simulink model "microgrid"  (R2021b)
settings: Solver=ode23tb  StartTime=0.0  StopTime=1  FixedStep=5e-6  RelTol=1e-3  EnableMultiTasking=on
PreLoadFcn:
  | % ---- microgrid : PreLoadFcn -------------------------------------
  | % Loads every base-workspace parameter this model needs.
  | %   SolarPVMPPTBoostData.mlx : PV array, boost converter, MPPT controller
  | %   microgridParams.m        : bus, battery, grid, drain, droop  (struct mg)
  | try
  |     mgDir = fileparts(which('microgrid'));
  |     if ~isempty(mgDir) && ~contains([path pathsep], [mgDir pathsep])
  |         addpath(mgDir);
  |     end
  |     evalc('SolarPVMPPTBoostData');
  |     microgridParams;
  |     clear mgDir
  |     disp('microgrid: parameters loaded (SolarPVMPPTBoostData + microgridParams).');
  | catch mgErr
  |     warning('microgrid:paramLoadFailed', ...
  |             'Could not load model parameters: %s', mgErr.message);
  |     clear mgErr
  | end
values from neighbouring files (symbols this model uses):
  mg = evalin('base','mg')    [microgridCheck.m]    (also in microgridParams.m = struct(); microgridScenario.m)
undefined symbols (not defined in the file or in its folder): boostController, dcVoltage, Ion, Lithium, sensor, solarPanel, solarPlant
libraries: powerlib_extras x46, fl_lib x12, simulink x8, nesl_utility x8, spsSeriesRLCBranchLib x7, spsCurrentMeasurementLib x7, spsGroundLib x6, spsVoltageMeasurementLib x6, spsIGBTDiodeLib x4, spsVariableResistorLib x4, slpidlib x4, ee_lib x3
(part 2 of 3)

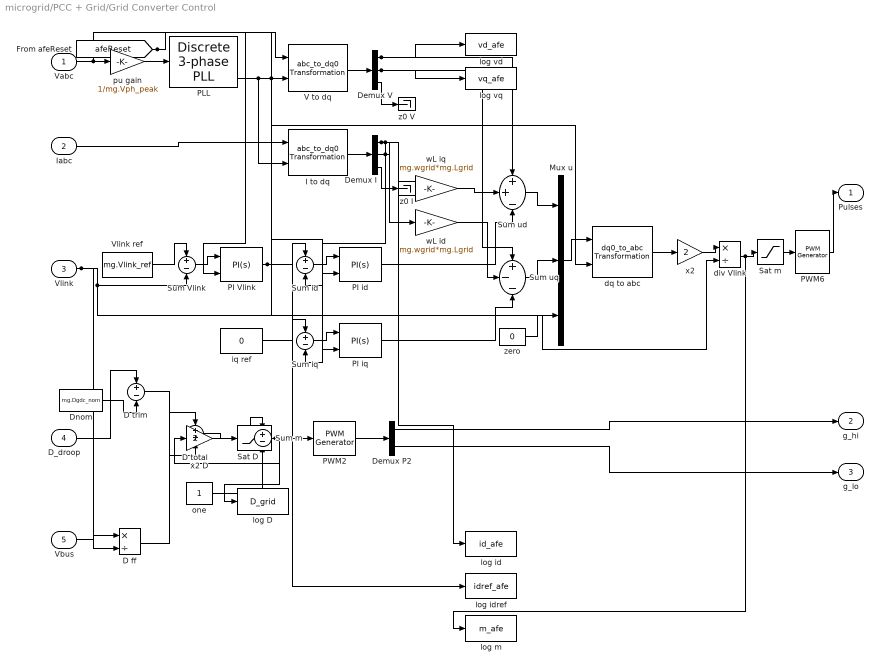
== system microgrid/PCC + Grid/Grid Converter Control ==
  Vabc : Inport
  Iabc : Inport  Port=2
  Vlink : Inport  Port=3
  D_droop : Inport  Port=4
  Vbus : Inport  Port=5
  D ff : Product  Inputs=*/
  D total : Sum
  D trim : Sum  Inputs=+-
  Demux I : Demux  Outputs=3
  Demux P2 : Demux  Outputs=2
  Demux V : Demux  Outputs=3
  Dnom : Constant  Value=mg.Dgdc_nom
  I to dq : powerlib_extras/Measurements/abc_to_dq0 Transformation
      settings: SourceProductBaseCode=PS
  Mux u : Mux  Inputs=3
  PI Vlink : slpidlib/PID Controller  Controller=PI  Form=Parallel  TimeDomain=Continuous-time  UseExternalTs=off  SampleTime=-1  IntegratorMethod=Forward Euler  FilterMethod=Forward Euler  ControllerParametersSource=internal  P=mg.Kp_v_afe  I=mg.Ki_v_afe  D=0  UseFilter=on  N=100  TunerSelectOption=Transfer Function Based (PID Tuner App)  InitialConditionSource=internal  InitialConditionForIntegrator=0  InitialConditionForFilter=0  DifferentiatorICPrevScaledInput=0  ExternalReset=level  TrackingMode=off  Kt=1  LimitOutput=on  SatLimitsSource=internal  UpperSaturationLimit=mg.Id_max  LowerSaturationLimit=-mg.Id_max  LinearizeAsGain=on  AntiWindupMode=clamping  Kb=1  POutMin=[]  POutMax=[]  IOutMin=[]  IOutMax=[]  DOutMin=[]  DOutMax=[]  NOutMin=[]  NOutMax=[]  SumOutMin=[]  SumOutMax=[]  SaturationOutMin=[]  SaturationOutMax=[]  PParamMin=[]  PParamMax=[]  IParamMin=[]  IParamMax=[]  DParamMin=[]  DParamMax=[]  NParamMin=[]  NParamMax=[]  KbParamMin=[]  KbParamMax=[]  KtParamMin=[]  KtParamMax=[]  KbOutMin=[]  KbOutMax=[]  KtOutMin=[]  KtOutMax=[]  IntegratorOutMin=[]  IntegratorOutMax=[]  FilterOutMin=[]  FilterOutMax=[]  SumI1OutMin=[]  SumI1OutMax=[]  SumI2OutMin=[]  SumI2OutMax=[]  SumI3OutMin=[]  SumI3OutMax=[]  SumI4OutMin=[]  SumI4OutMax=[]  SumDOutMin=[]  SumDOutMax=[]  DifferentiatorOutMin=[]  DifferentiatorOutMax=[]  FilterDiffOutCoefMin=[]  FilterDiffOutCoefMax=[]  ReciprocalOutMin=[]  ReciprocalOutMax=[]  SumDenOutMin=[]  SumDenOutMax=[]  SumNumOutMin=[]  SumNumOutMax=[]  DivideOutMin=[]  DivideOutMax=[]  UdiffTsProdOutMin=[]  UdiffTsProdOutMax=[]  NTsProdOutMin=[]  NTsProdOutMax=[]  UintegralTsProdOutMin=[]  UintegralTsProdOutMax=[]  UngainTsProdOutMin=[]  UngainTsProdOutMax=[]  FilterDenConstantOutDataTypeStr=Inherit: Inherit via back propagation  FilterDenConstantOutMin=[]  FilterDenConstantOutMax=[]  PCopyOutDataTypeStr=Inherit: Inherit via back propagation  PCopyOutMin=[]  PCopyOutMax=[]  NCopyOutDataTypeStr=Inherit: Inherit via back propagation  NCopyOutMin=[]  NCopyOutMax=[]  IntegratorContinuousStateAttributes=''  IntegratorStateMustResolveToSignalObject=off  IntegratorRTWStateStorageClass=Auto  FilterContinuousStateAttributes=''  FilterStateMustResolveToSignalObject=off  FilterRTWStateStorageClass=Auto  ParallelPVariant=InternalParameters  IdealPVariant=Disabled  IVariant=InternalParameters  DVariant=Disabled  IntegratorVariant=Continuous  SatVariant=Enabled  AWVariant=ContClampingParallel  PCopyVariant=Disabled  TRVariant=Disabled  FdbkBlocksVariant=Forward  IdealPFdbkVariant=Disabled  SatFdbkVariant=Disabled  DerivativeFilterVariant=Disabled  NVariant=Disabled  NCopyVariant=Disabled_SignalSpec  FilterICVariant=Disabled  IntegratorICVariant=InternalICs  ExternalResetVariant=ExternalReset  TRSumVariant=Passthrough  SumFdbkVariant=Disabled  SumVariant=Sum_PI  TsampFilterVariant=InternalTs  TsampNgainVariant=Passthrough  TsampIntegralVariant=Passthrough  ExternalSaturationOutDataTypeStr=Inherit: Same as second input
  PI id : slpidlib/PID Controller  Controller=PI  Form=Parallel  TimeDomain=Continuous-time  UseExternalTs=off  SampleTime=-1  IntegratorMethod=Forward Euler  FilterMethod=Forward Euler  ControllerParametersSource=internal  P=mg.Kp_i_afe  I=mg.Ki_i_afe  D=0  UseFilter=on  N=100  TunerSelectOption=Transfer Function Based (PID Tuner App)  InitialConditionSource=internal  InitialConditionForIntegrator=0  InitialConditionForFilter=0  DifferentiatorICPrevScaledInput=0  ExternalReset=level  TrackingMode=off  Kt=1  LimitOutput=on  SatLimitsSource=internal  UpperSaturationLimit=mg.Vph_peak  LowerSaturationLimit=-mg.Vph_peak  LinearizeAsGain=on  AntiWindupMode=clamping  Kb=1  POutMin=[]  POutMax=[]  IOutMin=[]  IOutMax=[]  DOutMin=[]  DOutMax=[]  NOutMin=[]  NOutMax=[]  SumOutMin=[]  SumOutMax=[]  SaturationOutMin=[]  SaturationOutMax=[]  PParamMin=[]  PParamMax=[]  IParamMin=[]  IParamMax=[]  DParamMin=[]  DParamMax=[]  NParamMin=[]  NParamMax=[]  KbParamMin=[]  KbParamMax=[]  KtParamMin=[]  KtParamMax=[]  KbOutMin=[]  KbOutMax=[]  KtOutMin=[]  KtOutMax=[]  IntegratorOutMin=[]  IntegratorOutMax=[]  FilterOutMin=[]  FilterOutMax=[]  SumI1OutMin=[]  SumI1OutMax=[]  SumI2OutMin=[]  SumI2OutMax=[]  SumI3OutMin=[]  SumI3OutMax=[]  SumI4OutMin=[]  SumI4OutMax=[]  SumDOutMin=[]  SumDOutMax=[]  DifferentiatorOutMin=[]  DifferentiatorOutMax=[]  FilterDiffOutCoefMin=[]  FilterDiffOutCoefMax=[]  ReciprocalOutMin=[]  ReciprocalOutMax=[]  SumDenOutMin=[]  SumDenOutMax=[]  SumNumOutMin=[]  SumNumOutMax=[]  DivideOutMin=[]  DivideOutMax=[]  UdiffTsProdOutMin=[]  UdiffTsProdOutMax=[]  NTsProdOutMin=[]  NTsProdOutMax=[]  UintegralTsProdOutMin=[]  UintegralTsProdOutMax=[]  UngainTsProdOutMin=[]  UngainTsProdOutMax=[]  FilterDenConstantOutDataTypeStr=Inherit: Inherit via back propagation  FilterDenConstantOutMin=[]  FilterDenConstantOutMax=[]  PCopyOutDataTypeStr=Inherit: Inherit via back propagation  PCopyOutMin=[]  PCopyOutMax=[]  NCopyOutDataTypeStr=Inherit: Inherit via back propagation  NCopyOutMin=[]  NCopyOutMax=[]  IntegratorContinuousStateAttributes=''  IntegratorStateMustResolveToSignalObject=off  IntegratorRTWStateStorageClass=Auto  FilterContinuousStateAttributes=''  FilterStateMustResolveToSignalObject=off  FilterRTWStateStorageClass=Auto  ParallelPVariant=InternalParameters  IdealPVariant=Disabled  IVariant=InternalParameters  DVariant=Disabled  IntegratorVariant=Continuous  SatVariant=Enabled  AWVariant=ContClampingParallel  PCopyVariant=Disabled  TRVariant=Disabled  FdbkBlocksVariant=Forward  IdealPFdbkVariant=Disabled  SatFdbkVariant=Disabled  DerivativeFilterVariant=Disabled  NVariant=Disabled  NCopyVariant=Disabled_SignalSpec  FilterICVariant=Disabled  IntegratorICVariant=InternalICs  ExternalResetVariant=ExternalReset  TRSumVariant=Passthrough  SumFdbkVariant=Disabled  SumVariant=Sum_PI  TsampFilterVariant=InternalTs  TsampNgainVariant=Passthrough  TsampIntegralVariant=Passthrough  ExternalSaturationOutDataTypeStr=Inherit: Same as second input
  PI iq : slpidlib/PID Controller  Controller=PI  Form=Parallel  TimeDomain=Continuous-time  UseExternalTs=off  SampleTime=-1  IntegratorMethod=Forward Euler  FilterMethod=Forward Euler  ControllerParametersSource=internal  P=mg.Kp_i_afe  I=mg.Ki_i_afe  D=0  UseFilter=on  N=100  TunerSelectOption=Transfer Function Based (PID Tuner App)  InitialConditionSource=internal  InitialConditionForIntegrator=0  InitialConditionForFilter=0  DifferentiatorICPrevScaledInput=0  ExternalReset=level  TrackingMode=off  Kt=1  LimitOutput=on  SatLimitsSource=internal  UpperSaturationLimit=mg.Vph_peak  LowerSaturationLimit=-mg.Vph_peak  LinearizeAsGain=on  AntiWindupMode=clamping  Kb=1  POutMin=[]  POutMax=[]  IOutMin=[]  IOutMax=[]  DOutMin=[]  DOutMax=[]  NOutMin=[]  NOutMax=[]  SumOutMin=[]  SumOutMax=[]  SaturationOutMin=[]  SaturationOutMax=[]  PParamMin=[]  PParamMax=[]  IParamMin=[]  IParamMax=[]  DParamMin=[]  DParamMax=[]  NParamMin=[]  NParamMax=[]  KbParamMin=[]  KbParamMax=[]  KtParamMin=[]  KtParamMax=[]  KbOutMin=[]  KbOutMax=[]  KtOutMin=[]  KtOutMax=[]  IntegratorOutMin=[]  IntegratorOutMax=[]  FilterOutMin=[]  FilterOutMax=[]  SumI1OutMin=[]  SumI1OutMax=[]  SumI2OutMin=[]  SumI2OutMax=[]  SumI3OutMin=[]  SumI3OutMax=[]  SumI4OutMin=[]  SumI4OutMax=[]  SumDOutMin=[]  SumDOutMax=[]  DifferentiatorOutMin=[]  DifferentiatorOutMax=[]  FilterDiffOutCoefMin=[]  FilterDiffOutCoefMax=[]  ReciprocalOutMin=[]  ReciprocalOutMax=[]  SumDenOutMin=[]  SumDenOutMax=[]  SumNumOutMin=[]  SumNumOutMax=[]  DivideOutMin=[]  DivideOutMax=[]  UdiffTsProdOutMin=[]  UdiffTsProdOutMax=[]  NTsProdOutMin=[]  NTsProdOutMax=[]  UintegralTsProdOutMin=[]  UintegralTsProdOutMax=[]  UngainTsProdOutMin=[]  UngainTsProdOutMax=[]  FilterDenConstantOutDataTypeStr=Inherit: Inherit via back propagation  FilterDenConstantOutMin=[]  FilterDenConstantOutMax=[]  PCopyOutDataTypeStr=Inherit: Inherit via back propagation  PCopyOutMin=[]  PCopyOutMax=[]  NCopyOutDataTypeStr=Inherit: Inherit via back propagation  NCopyOutMin=[]  NCopyOutMax=[]  IntegratorContinuousStateAttributes=''  IntegratorStateMustResolveToSignalObject=off  IntegratorRTWStateStorageClass=Auto  FilterContinuousStateAttributes=''  FilterStateMustResolveToSignalObject=off  FilterRTWStateStorageClass=Auto  ParallelPVariant=InternalParameters  IdealPVariant=Disabled  IVariant=InternalParameters  DVariant=Disabled  IntegratorVariant=Continuous  SatVariant=Enabled  AWVariant=ContClampingParallel  PCopyVariant=Disabled  TRVariant=Disabled  FdbkBlocksVariant=Forward  IdealPFdbkVariant=Disabled  SatFdbkVariant=Disabled  DerivativeFilterVariant=Disabled  NVariant=Disabled  NCopyVariant=Disabled_SignalSpec  FilterICVariant=Disabled  IntegratorICVariant=InternalICs  ExternalResetVariant=ExternalReset  TRSumVariant=Passthrough  SumFdbkVariant=Disabled  SumVariant=Sum_PI  TsampFilterVariant=InternalTs  TsampNgainVariant=Passthrough  TsampIntegralVariant=Passthrough  ExternalSaturationOutDataTypeStr=Inherit: Same as second input
  PLL : powerlib_extras/Discrete  Control Blocks/Discrete 3-phase PLL  Fmin=0.8*mg.fgrid  Par_Init=[0 mg.fgrid]  ParK=[ 180 3200 1 ]  Ts=mg.Ts_pll  AGC=on
      settings: SourceProductBaseCode=PS
  PWM2 : powerlib_extras/Control  Blocks/PWM Generator  GeneratorMode="1-arm  bridge (2 pulses)"  Fc=mg.fsw_gdc  Internal=off  mIndex=0.4  Freq=mg.fgrid  Phase=0
      settings: SourceProductBaseCode=PS
  PWM6 : powerlib_extras/Control  Blocks/PWM Generator  GeneratorMode="3-arm  bridge (6 pulses)"  Fc=mg.fsw_afe  Internal=off  mIndex=0.4  Freq=mg.fgrid  Phase=0
      settings: SourceProductBaseCode=PS
  Sat D : Saturate  UpperLimit=mg.Dgdc_max  LowerLimit=mg.Dgdc_min
  Sat m : Saturate  UpperLimit=1  LowerLimit=-1
  Sum Vlink : Sum  Inputs=+-
  Sum id : Sum  Inputs=+-
  Sum iq : Sum  Inputs=+-
  Sum m : Sum  Inputs=+-
  Sum ud : Sum  Inputs=++-
  Sum uq : Sum  Inputs=+--
  V to dq : powerlib_extras/Measurements/abc_to_dq0 Transformation
      settings: SourceProductBaseCode=PS
  Vlink ref : Constant  Value=mg.Vlink_ref
  div Vlink : Product  Inputs=*/
  dq to abc : powerlib_extras/Measurements/dq0_to_abc Transformation
      settings: SourceProductBaseCode=PS
  iq ref : Constant  Value=0
  log D : ToWorkspace  VariableName=D_grid  SampleTime=-1
      settings: Decimation=20
  log id : ToWorkspace  VariableName=id_afe  SampleTime=-1
      settings: Decimation=20
  log idref : ToWorkspace  VariableName=idref_afe  SampleTime=-1
      settings: Decimation=20
  log m : ToWorkspace  VariableName=m_afe  SampleTime=-1
      settings: Decimation=20
  log vd : ToWorkspace  VariableName=vd_afe  SampleTime=-1
      settings: Decimation=20
  log vq : ToWorkspace  VariableName=vq_afe  SampleTime=-1
      settings: Decimation=20
  one : Constant
  pu gain : Gain  Gain=1/mg.Vph_peak
  wL id : Gain  Gain=mg.wgrid*mg.Lgrid
  wL iq : Gain  Gain=mg.wgrid*mg.Lgrid
  x2 : Gain  Gain=2
  x2 D : Gain  Gain=2
  z0 I : Terminator
  z0 V : Terminator
  zero : Constant  Value=0
  Pulses : Outport
  g_hi : Outport  Port=2
  g_lo : Outport  Port=3
  wires:
  Vabc/1 -> pu gain/1, V to dq/1
  pu gain/1 -> PLL/1
  PLL/3 -> V to dq/2, dq to abc/2, I to dq/2
  Iabc/1 -> I to dq/1
  V to dq/1 -> Demux V/1
  I to dq/1 -> Demux I/1
  Vlink ref/1 -> Sum Vlink/1
  Vlink/1 -> Sum Vlink/2, div Vlink/2, D ff/2
  Sum Vlink/1 -> PI Vlink/1
  PI Vlink/1 -> Sum id/1, log idref/1
  Demux I/1 -> Sum id/2, wL id/1, log id/1
  iq ref/1 -> Sum iq/1
  Demux I/2 -> Sum iq/2, wL iq/1
  Sum id/1 -> PI id/1
  Sum iq/1 -> PI iq/1
  Demux V/1 -> Sum ud/1, log vd/1
  wL iq/1 -> Sum ud/2
  PI id/1 -> Sum ud/3
  Demux V/2 -> Sum uq/1, log vq/1
  wL id/1 -> Sum uq/2
  PI iq/1 -> Sum uq/3
  Sum ud/1 -> Mux u/1
  Sum uq/1 -> Mux u/2
  zero/1 -> Mux u/3
  Mux u/1 -> dq to abc/1
  dq to abc/1 -> x2/1
  x2/1 -> div Vlink/1
  div Vlink/1 -> Sat m/1, log m/1
  Sat m/1 -> PWM6/1
  PWM6/1 -> Pulses/1
  x2 D/1 -> Sum m/1
  one/1 -> Sum m/2
  Sum m/1 -> PWM2/1
  PWM2/1 -> Demux P2/1
  Demux P2/1 -> g_hi/1
  Demux P2/2 -> g_lo/1
  Vbus/1 -> D ff/1
  D_droop/1 -> D trim/1
  Dnom/1 -> D trim/2
  D ff/1 -> D total/1
  D trim/1 -> D total/2
  D total/1 -> Sat D/1
  Sat D/1 -> x2 D/1, log D/1
  Demux V/3 -> z0 V/1
  Demux I/3 -> z0 I/1
  [afeReset] -> PI Vlink/2, PI id/2, PI iq/2

== system microgrid/PV + Boost/AC Current Sensor2 ==
  Current Sensor : fl_lib/Electrical/Electrical Sensors/Current Sensor
  PS-Simulink Converter : nesl_utility/PS-Simulink Converter  PhysicalDomain=network_engine_domain  SubClassName=ps_output  LeftPortType=input  RightPortType=output  PseudoPeriodic=off  Frequencies=[]  Unit=1  AffineConversion=off
      settings: SourceProductBaseCode=PW,SS
  Sensor dynamics : TransferFcn  Numerator=1  Denominator=[1/sensor.samplingFreq 1]
  - : PMIOPort  Side=Left
  + : PMIOPort  Port=2  Side=Right
  tag scope: Iload=global
  wires:
  PS-Simulink Converter/1 -> Sensor dynamics/1
  Sensor dynamics/1 -> [Iload]
  connections:
  Current Sensor/RConn1 -- PS-Simulink Converter/LConn1
  +/RConn1 -- Current Sensor/LConn1
  Current Sensor/RConn2 -- -/RConn1

== system microgrid/PV + Boost/Boost Converter ==
  m : Inport
  AC Current Sensor1 : Subsystem
      mask Display: disp('i');
  DC Bus Capacitor : fl_lib/Electrical/Electrical Elements/Capacitor  c=mg.Cbus F  r=1e-6 Ohm  g=0 1/Ohm  i_specify=off  i_priority=None  i=0 A  i_nominal_specify=off  i_nominal_unit=A  i_nominal_value=1  v_specify=off  v_priority=None  v=0 V  v_nominal_specify=off  v_nominal_unit=V  v_nominal_value=1  vc_specify=on  vc_priority=High  vc=mg.Vbus_nom V  vc_nominal_specify=off  vc_nominal_unit=V  vc_nominal_value=1
  Diode : fl_lib/Electrical/Electrical Elements/Diode  Vf=0.6 V  Ron=0.3 Ohm  Goff=1e-8 1/Ohm  i_specify=off  i_priority=None  i=0 A  i_nominal_specify=off  i_nominal_unit=A  i_nominal_value=1  v_specify=off  v_priority=None  v=0 V  v_nominal_specify=off  v_nominal_unit=V  v_nominal_value=1
  Gain : Gain  Gain=5
  "IGBT (Ideal, Switching)1" : ee_lib/Semiconductors & Converters/IGBT (Ideal, Switching)  Vf=0.8 V  Ron=0.001 Ohm  Goff=1e-5 1/Ohm  Vth=2.5 V  diode_param=1  diode_Vf=0.8 V  diode_Ron=0.001 Ohm  diode_Goff=1e-5 1/Ohm  diode_C=50e-9 F  diode_iRM=-235 A  diode_iF=300 A  diode_idot=-50 A/us  diode_trr_param=1  diode_trr_factor=3  diode_trr=15 us  diode_Qrr=1500 s*uA  thermal_loss_option=ee.enum.converters.thermalLossOption.constantvalues  Von_data=[0, .1, .6, .8, 1, 1.3, 1.6, 2, 2.4; 0, .1, .7, 1, 1.2, 1.5, 1.9, 2.4, 2.8] V  Tj=[298.15, 398.15] K  Iout_data=[0, .1, 1, 5, 10, 20, 40, 70, 100] A  Eon_data=[0, .0024, .024, .12, .2, .48, 1.04, 2.16, 3.24; 0, .003, .03, .15, .25, .6, 1.3, 2.7, 4.05] * 1e-3 J  Eoff_data=[0, .0007, .0066, .033, .066, .17, .33, .83, 1.5; 0, .001, .01, .05, .1, .25, .5, 1.2, 2.2] * 1e-3 J  Tj_loss=[298.15, 398.15] K  Iout_data_loss=[0, .1, 1, 5, 10, 20, 40, 70, 100] A  Eon_scalar=22.86e-3 J  Eoff_scalar=17.14e-3 J  Voff=300 V  Iout_scalar=600 A  diodeModelType=ee.enum.converters.diodeModelType.pwl  diodeTableType=ee.enum.diode.tableType.IfMat  diode_IfMat=[.07, .12, .19, 1.75, 4.24, 7.32, 11.2; .16, .3, .72, 2.14, 4.02, 6.35, 9.12] A  diode_VfMat=[.9, 1.15, 1.25, 1.5, 1.75, 2.17, 2.6, 2.85; .58, .68, .75, 1.1, 1.38, 1.77, 2.27, 2.7] V  diode_TjVec=[25, 125] degC  diode_VfVec=[.5, .7, .9, 1.3, 1.7, 2.1, 2.5] V  diode_IfVec=[.1, .2, .5, 1, 2, 4, 7, 10] A  diode_Vr=-600 V  diode_Ls=150 nH  diode_Erec=0.03 J  thermal_network_parameterization=ee.enum.thermalNetworkTopology.external  Rth=[.08, .5] K/W  Rth_Cauer=[.08, .1, .5] K/W  Rth_Foster=[.08, .14, .22, .16] K/W  thermal_mass_parameterization=ee.enum.thermalNetwork.timeconstant  thermal_mass=[.01, .5] J/K  thermal_mass_Cauer=[.01, .1, .5] J/K  thermal_mass_Foster=[.001, .005, .05, .5] J/K  thermal_time_constant=[.001, .2] s  thermal_time_constant_Cauer=[.001, .1, .2] s  thermal_time_constant_Foster=[7e-05, .0007, .01, .08] s  thermal_mass_initial_temperatures=[25, 25] degC  thermal_mass_initial_temperatures_Cauer=[25, 25, 25] degC  junction_thermal_mass=0.01 J/K  steadyState_Foster=simscape.enum.onoff.on  Tvec_initial_Foster=[25, 25, 25, 25] degC  no_thermal_network=0  junction_temperature_specify=off  junction_temperature_priority=None  junction_temperature=25 degC  junction_temperature_nominal_specify=off  junction_temperature_nominal_unit=degC  junction_temperature_nominal_value=1  vT_specify=off  vT_priority=None  vT=0 V  vT_nominal_specify=off  vT_nominal_unit=V  vT_nominal_value=1  Qj_specify=off  Qj_priority=None  Qj=0 W  Qj_nominal_specify=off  Qj_nominal_unit=W  Qj_nominal_value=1
  MPPT Inductor : ee_lib/Passive/Inductor  l=boost.inductor H  L_tol=5  enable_L_tol=0  tol_distribution=1  nSigma=4  r=boost.inductorResistance Ohm  g=1e-9 1/Ohm  enable_operating_limits=0  operating_limit_action=2  max_working_current=1 A  power_rating=1 W  enable_faults=0  fault_action=simscape.enum.assert.action.none  lambdaPercent=50  k_faulted=0.9999  turnsShort=0  openCct=0  groundShort=0  groundShortG=0 1/Ohm  tau_fault=1e-3 s  enable_temporal_fault=0  t_fault=1 s  enable_behavioral_fault=0  max_permissible_voltage=100 V  n_fail_on_voltage=1  max_permissible_current=1 A  t_fail_on_current=1 s  i_L_specify=on  i_L_priority=High  i_L=0 A  i_L_nominal_specify=off  i_L_nominal_unit=A  i_L_nominal_value=1
  Simulink-PS Converter : nesl_utility/Simulink-PS Converter  PhysicalDomain=network_engine_domain  SubClassName=ps_input  LeftPortType=input  RightPortType=output  PseudoPeriodic=off  Frequencies=[]  NoiseDistribution=none  NoiseParameters=[]  Unit=1  AffineConversion=off  FilteringAndDerivatives=provide  SimscapeFilterOrder=1  InputFilterTimeConstant=0.001  UdotUserProvided=0
      settings: SourceProductBaseCode=PW,SS
  + : PMIOPort  Side=Left
  P : PMIOPort  Port=2  Side=Right
  N : PMIOPort  Port=3  Side=Right
  - : PMIOPort  Port=4  Side=Left
  wires:
  m/1 -> Gain/1
  Gain/1 -> Simulink-PS Converter/1
  connections:
  MPPT Inductor/LConn1 -- AC Current Sensor1/LConn1
  N/RConn1 -- DC Bus Capacitor/RConn1 -- "IGBT (Ideal, Switching)1"/RConn2 -- -/RConn1
  AC Current Sensor1/RConn1 -- +/RConn1
  "IGBT (Ideal, Switching)1"/LConn1 -- Simulink-PS Converter/RConn1
  MPPT Inductor/RConn1 -- "IGBT (Ideal, Switching)1"/RConn1 -- Diode/LConn1
  DC Bus Capacitor/LConn1 -- Diode/RConn1 -- P/RConn1

== system microgrid/PV + Boost/DC Current Sensor ==
  Current Sensor : fl_lib/Electrical/Electrical Sensors/Current Sensor
      settings: LogSimulationData=on
  PS-Simulink Converter : nesl_utility/PS-Simulink Converter  PhysicalDomain=network_engine_domain  SubClassName=ps_output  LeftPortType=input  RightPortType=output  PseudoPeriodic=off  Frequencies=[]  Unit=1  AffineConversion=off
      settings: SourceProductBaseCode=PW,SS
  Sensor dynamics : TransferFcn  Numerator=1  Denominator=[1/sensor.samplingFreq 1]
  - : PMIOPort  Side=Left
  + : PMIOPort  Port=2  Side=Right
  tag scope: Ipv=global
  wires:
  PS-Simulink Converter/1 -> Sensor dynamics/1
  Sensor dynamics/1 -> [Ipv]
  connections:
  Current Sensor/RConn2 -- -/RConn1
  +/RConn1 -- Current Sensor/LConn1
  Current Sensor/RConn1 -- PS-Simulink Converter/LConn1

== system microgrid/PV + Boost/DC Output Voltage Sensor ==
  PS-Simulink Converter : nesl_utility/PS-Simulink Converter  PhysicalDomain=network_engine_domain  SubClassName=ps_output  LeftPortType=input  RightPortType=output  PseudoPeriodic=off  Frequencies=[]  Unit=1  AffineConversion=off
      settings: SourceProductBaseCode=PW,SS
  Sensor dynamics : TransferFcn  Numerator=1  Denominator=[1/sensor.samplingFreq 1]
  Voltage Sensor : fl_lib/Electrical/Electrical Sensors/Voltage Sensor
  - : PMIOPort  Side=Left
  + : PMIOPort  Port=2  Side=Right
  tag scope: Vo=global
  wires:
  PS-Simulink Converter/1 -> Sensor dynamics/1
  Sensor dynamics/1 -> [Vo]
  connections:
  Voltage Sensor/RConn2 -- -/RConn1
  Voltage Sensor/RConn1 -- PS-Simulink Converter/LConn1
  Voltage Sensor/LConn1 -- +/RConn1

== system microgrid/PV + Boost/DC Voltage Sensor ==
  PS-Simulink Converter : nesl_utility/PS-Simulink Converter  PhysicalDomain=network_engine_domain  SubClassName=ps_output  LeftPortType=input  RightPortType=output  PseudoPeriodic=off  Frequencies=[]  Unit=1  AffineConversion=off
      settings: SourceProductBaseCode=PW,SS
  Sensor dynamics : TransferFcn  Numerator=1  Denominator=[1/sensor.samplingFreq 1]
  Voltage Sensor : fl_lib/Electrical/Electrical Sensors/Voltage Sensor
      settings: LogSimulationData=on
  - : PMIOPort  Side=Left
  + : PMIOPort  Port=2  Side=Right
  tag scope: Vpv=global
  wires:
  PS-Simulink Converter/1 -> Sensor dynamics/1
  Sensor dynamics/1 -> [Vpv]
  connections:
  Voltage Sensor/LConn1 -- +/RConn1
  Voltage Sensor/RConn1 -- PS-Simulink Converter/LConn1
  Voltage Sensor/RConn2 -- -/RConn1

== system microgrid/PV + Boost/Irradiance ==
  " " : Constant
  Solar Irradiance W/m2 : Gain  Gain=150
  Irad : Outport
  wires:
  " "/1 -> Solar Irradiance W/m2/1
  Solar Irradiance W/m2/1 -> Irad/1

== system microgrid/PV + Boost/Monitoring ==
  "  " : TransferFcn  Denominator=[1e-2 1]
  Load Power : TransferFcn  Denominator=[1e-2 1]
  Load Power1 : TransferFcn  Denominator=[1e-2 1]
  Product : Product
  Product1 : Product
  Terminator1 : Terminator
  Terminator2 : Terminator
  Terminator7 : Terminator
  W2kW : Gain  Gain=1e-3
  gain : Gain  Gain=1e-3
  wires:
  [Vpv] -> Product/2  "Vpv(V)"
  Load Power/1 -> gain/1
  Product1/1 -> Load Power/1  "P(W)"
  [Iload] -> Product1/1
  "  "/1 -> Terminator1/1  "Solar PV Power (kW)"
  [Ipv] -> Product/1
  [Vo] -> Product1/2, Load Power1/1
  Product/1 -> W2kW/1  "P(W)"
  gain/1 -> Terminator2/1  "Load Power (kW)"
  W2kW/1 -> "  "/1
  Load Power1/1 -> Terminator7/1  "DC Bus Voltage (V)"

== system microgrid/PV + Boost/PV Control ==
  Vo : Inport
  Ipv : Inport  Port=2
  Vpv : Inport  Port=3
  IL : Inport  Port=4
  Vref : Inport  Port=5
  Constant Voltage : Subsystem
  Maximum Power Point : Subsystem
  Merge : Merge
  PV Mode : Subsystem
  Terminator : Terminator
  Gate : Outport
  wires:
  Merge/1 -> Gate/1
  Vo/1 -> Maximum Power Point/2("Vo "), Constant Voltage/3("Vo ")
  Maximum Power Point/1(Gmpp) -> Merge/2
  [VoltCtrl] -> Constant Voltage/Enable
  IL/1 -> Maximum Power Point/1("IL "), Constant Voltage/4(IL)
  Vpv/1 -> Maximum Power Point/3(Vpv), Constant Voltage/2(Vpv)
  Ipv/1 -> Maximum Power Point/4(Ipv)
  Constant Voltage/1(G) -> Merge/1
  Maximum Power Point/2(Vmpp) -> Terminator/1
  [pvMPPT] -> Maximum Power Point/Enable
  PV Mode/1(MPPT) -> [pvMPPT]
  PV Mode/2(VoltCtrl) -> [VoltCtrl]
  Vref/1 -> Constant Voltage/1(Vconst)

== system microgrid/PV + Boost/Solar Plant ==
  Current-Controlled Current Source- Scale panel current to Np parallel strings : fl_lib/Electrical/Electrical Sources/Current-Controlled Current Source  K=-1*(solarPlant.numParallelPanel-1)  i1_specify=off  i1_priority=None  i1=0 A  i1_nominal_specify=off  i1_nominal_unit=A  i1_nominal_value=1  i2_specify=off  i2_priority=None  i2=0 A  i2_nominal_specify=off  i2_nominal_unit=A  i2_nominal_value=1
      settings: SourceProductBaseCode=SS  InternalSimscapePortConfiguration="{\"Bottom\":[],\"Left\":[{\"id\":\"p1\",\"label\":\"+\",\"type\":\"foundation.electrical.electrical\"},{\"id\":\"head\",\"label\":\"\",\"type\":\"foundation.electrical.electrical\"}],\"Right\":[{\"id\":\"n1\",\"label\":\"-\",\"type\":\"foundation.electrical.electrical\"},{\"id\":\"tail\",\"label\":\"\",\"type\":\"foundation.electrical.electrical\"}],\"Top\":[]}"
  Solar Panel : Subsystem  mask(Solar Panel){}
      mask help: Models a solar panel using a parallel-connected sting of solar cells. The solar cell strings are modeled using a single Solar Cell block from the Simscape(TM) Electrical(TM) Sources library.
      mask Display: image('SolarPanelValidationIcon.jpg')
  Voltage-Controlled Voltage Source - Scale panel voltage to Ns series panel : fl_lib/Electrical/Electrical Sources/Voltage-Controlled Voltage Source  K=-1*(solarPlant.numSeriesPanel-1)  v1_specify=off  v1_priority=None  v1=0 V  v1_nominal_specify=off  v1_nominal_unit=V  v1_nominal_value=1  v2_specify=off  v2_priority=None  v2=0 V  v2_nominal_specify=off  v2_nominal_unit=V  v2_nominal_value=1
      settings: SourceProductBaseCode=SS  InternalSimscapePortConfiguration="{\"Bottom\":[],\"Left\":[{\"id\":\"p1\",\"label\":\"+\",\"type\":\"foundation.electrical.electrical\"},{\"id\":\"p2\",\"label\":\"+\",\"type\":\"foundation.electrical.electrical\"}],\"Right\":[{\"id\":\"n1\",\"label\":\"-\",\"type\":\"foundation.electrical.electrical\"},{\"id\":\"n2\",\"label\":\"-\",\"type\":\"foundation.electrical.electrical\"}],\"Top\":[]}"
  + : PMIOPort  Side=Right
  Irradiance : PMIOPort  Port=2  Side=Left
  - : PMIOPort  Port=3  Side=Right
  connections:
  Voltage-Controlled Voltage Source - Scale panel voltage to Ns series panel/RConn2 -- Voltage-Controlled Voltage Source - Scale panel voltage to Ns series panel/RConn1 -- Solar Panel/RConn1
  Voltage-Controlled Voltage Source - Scale panel voltage to Ns series panel/LConn1 -- Current-Controlled Current Source- Scale panel current to Np parallel strings/LConn2 -- -/RConn1 -- Solar Panel/RConn2
  Current-Controlled Current Source- Scale panel current to Np parallel strings/RConn1 -- Current-Controlled Current Source- Scale panel current to Np parallel strings/RConn2 -- +/RConn1
  Current-Controlled Current Source- Scale panel current to Np parallel strings/LConn1 -- Voltage-Controlled Voltage Source - Scale panel voltage to Ns series panel/LConn2
  Solar Panel/LConn1 -- Irradiance/RConn1

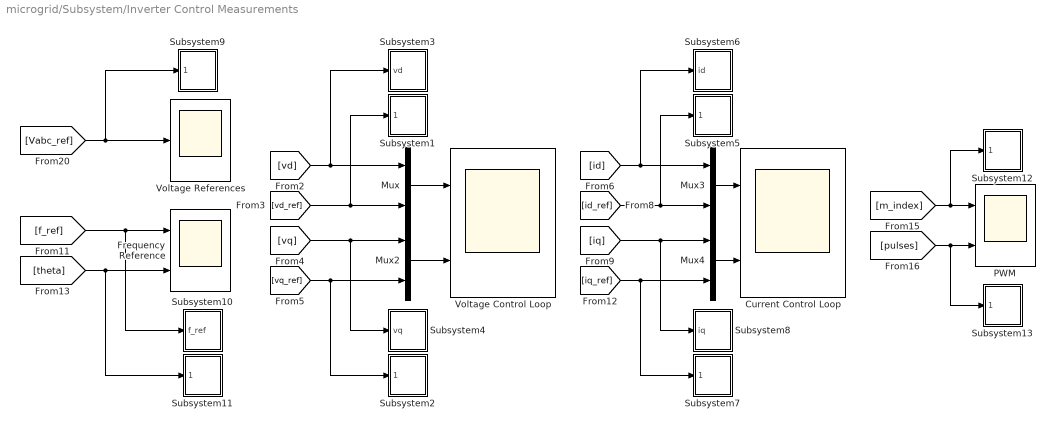
== system microgrid/Subsystem/Inverter Control Measurements ==
  Current Control Loop : Scope  NumInputPorts=2
  Frequency Reference : Scope  NumInputPorts=2
  Mux{,2..4} (4 alike) : Mux  Inputs=2
  PWM : Scope  NumInputPorts=2
  Subsystem1 : Subsystem
  Subsystem10 : Subsystem
  Subsystem11 : Subsystem
  Subsystem12 : Subsystem
  Subsystem13 : Subsystem
  Subsystem2 : Subsystem
  Subsystem3 : Subsystem
  Subsystem4 : Subsystem
  Subsystem5 : Subsystem
  Subsystem6 : Subsystem
  Subsystem7 : Subsystem
  Subsystem8 : Subsystem
  Subsystem9 : Subsystem
  Voltage Control Loop : Scope  NumInputPorts=2
  Voltage References : Scope
  wires:
  [vd] -> Mux/1, Subsystem3/1(vd)
  [vd_ref] -> Mux/2, Subsystem1/1(vd_ref)
  [vq] -> Mux2/1, Subsystem4/1(vq)
  [vq_ref] -> Mux2/2, Subsystem2/1(vq_ref)
  Mux/1 -> Voltage Control Loop/1
  Mux2/1 -> Voltage Control Loop/2
  [id] -> Mux3/1, Subsystem6/1(id)
  [id_ref] -> Mux3/2, Subsystem5/1(id_ref)
  [iq] -> Mux4/1, Subsystem8/1(iq)
  [iq_ref] -> Mux4/2, Subsystem7/1(iq_ref)
  [Vabc_ref] -> Voltage References/1, Subsystem9/1(Vabc_ref)
  Mux3/1 -> Current Control Loop/1
  Mux4/1 -> Current Control Loop/2
  [theta] -> Frequency Reference/2, Subsystem11/1(theta)
  [f_ref] -> Frequency Reference/1, Subsystem10/1(f_ref)
  [pulses] -> PWM/2, Subsystem13/1(pulses)
  [m_index] -> PWM/1, Subsystem12/1(m_index)

== system microgrid/Subsystem/Inverter Control Measurements1 ==
  Boost Converter Control MPPT : Scope  NumInputPorts=3
  wires:
  [Vref] -> Boost Converter Control MPPT/1
  [delta] -> Boost Converter Control MPPT/2
  [pulsos] -> Boost Converter Control MPPT/3

== system microgrid/Subsystem/Inverter Control Measurements2 ==
  Control Loops : Scope  NumInputPorts=2
  Mux : Mux  Inputs=2
  Mux2 : Mux  Inputs=2
  Switch Control : Scope  NumInputPorts=3
  wires:
  [Vdc] -> Mux/1
  [Vdc_ref] -> Mux/2
  [Ibat] -> Mux2/1
  [Ibat_ref] -> Mux2/2
  Mux/1 -> Control Loops/1
  Mux2/1 -> Control Loops/2
  [Sign] -> Switch Control/1
  [S1] -> Switch Control/2
  [S2] -> Switch Control/3

== system microgrid/Subsystem/Inverter Control Measurements3 ==
  PLL : Subsystem
  Subsystem : Subsystem
  wires:
  Subsystem/1(Vabc) -> PLL/1(Vabc)

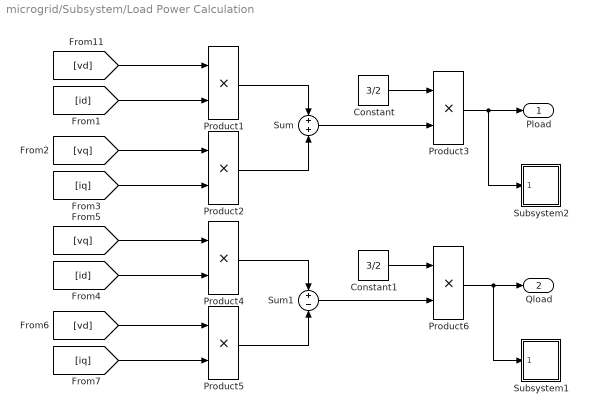
== system microgrid/Subsystem/Load Power Calculation ==
  Constant : Constant  Value=3/2
  Constant1 : Constant  Value=3/2
  Product{1..6} (6 alike) : Product  RndMeth=Zero
  Subsystem1 : Subsystem
  Subsystem2 : Subsystem
  Sum : Sum  Inputs=+|+
  Sum1 : Sum  Inputs=+|-
  Pload : Outport
  Qload : Outport  Port=2
  wires:
  [vd] -> Product1/1
  [id] -> Product1/2
  [vq] -> Product2/1
  [iq] -> Product2/2
  Product1/1 -> Sum/1
  Product2/1 -> Sum/2
  Sum/1 -> Product3/2
  Constant/1 -> Product3/1
  Product3/1 -> Pload/1, Subsystem2/1(Pload)
  [vq] -> Product4/1
  [id] -> Product4/2
  [vd] -> Product5/1
  [iq] -> Product5/2
  Product4/1 -> Sum1/1
  Product5/1 -> Sum1/2
  Sum1/1 -> Product6/2
  Constant1/1 -> Product6/1
  Product6/1 -> Qload/1, Subsystem1/1(Qacload)

== system microgrid/Subsystem/Subsystem ==
  Mux : Mux  Inputs=3
  Vabc : Outport
  wires:
  Mux/1 -> Vabc/1
  [Vab] -> Mux/1
  [Vbc] -> Mux/2
  [Vca] -> Mux/3

== system microgrid/Subsystem/Subsystem1 ==
  Pbus : Inport
  LPF vq11 : powerlib_extras/Discrete  Control Blocks/Discrete 1st-Order Filter  FilterType=Lowpass  Tc=10e-3  Ts=5e-6  Initialize=off  Vac_Init=[0.8 -25 60]  Vdc_Init=0  PlotResponse=off  param1=[1 100 0.1]
      settings: SourceProductBaseCode=PS
  To Workspace1 : ToWorkspace  VariableName=Pbus  SampleTime=-1
  To Workspace2 : ToWorkspace  VariableName=Pbus1  SampleTime=-1
  tag scope: Pbus=global
  wires:
  Pbus/1 -> [Pbus], To Workspace1/1, LPF vq11/1
  LPF vq11/1 -> To Workspace2/1

== system microgrid/Subsystem/Subsystem10 ==
  f : Inport
  LPF vq7 : powerlib_extras/Discrete  Control Blocks/Discrete 1st-Order Filter  FilterType=Lowpass  Tc=10e-3  Ts=5e-6  Initialize=off  Vac_Init=[0.8 -25 60]  Vdc_Init=0  PlotResponse=off  param1=[1 100 0.1]
      settings: SourceProductBaseCode=PS
  To Workspace1 : ToWorkspace  VariableName=fabc_real  SampleTime=-1
  To Workspace2 : ToWorkspace  VariableName=fabc_real_fil  SampleTime=-1
  Zero-Order Hold : ZeroOrderHold  SampleTime=5e-6
  wires:
  f/1 -> Zero-Order Hold/1
  LPF vq7/1 -> To Workspace2/1
  Zero-Order Hold/1 -> To Workspace1/1, LPF vq7/1

== system microgrid/Subsystem/Subsystem11 ==
  LPF vq{2..3,8..9} (4 alike) : powerlib_extras/Discrete  Control Blocks/Discrete 1st-Order Filter  FilterType=Lowpass  Tc=10e-3  Ts=5e-6  Initialize=off  Vac_Init=[0.8 -25 60]  Vdc_Init=0  PlotResponse=off  param1=[1 100 0.1]
      settings: SourceProductBaseCode=PS
  Load Measurements1 : Scope  NumInputPorts=2
  Load Measurements3 : Scope  NumInputPorts=2
  Load Power Calculation1 : Subsystem
  Load Power Calculation2 : Subsystem
  Load Powers1 : Scope  NumInputPorts=2
  Load Powers2 : Scope  NumInputPorts=2
  wires:
  [Vabc2] -> Load Measurements1/1
  [Iabc2] -> Load Measurements1/2
  Load Power Calculation1/1(Pload) -> LPF vq2/1
  Load Power Calculation1/2(Qload) -> LPF vq3/1
  LPF vq2/1 -> Load Powers1/1
  LPF vq3/1 -> Load Powers1/2
  [Vabc3] -> Load Measurements3/1
  [Iabc3] -> Load Measurements3/2
  Load Power Calculation2/1(Pload) -> LPF vq8/1
  Load Power Calculation2/2(Qload) -> LPF vq9/1
  LPF vq8/1 -> Load Powers2/1
  LPF vq9/1 -> Load Powers2/2

== system microgrid/Subsystem/Subsystem3 ==
  Pdc : Inport
  LPF vq7 : powerlib_extras/Discrete  Control Blocks/Discrete 1st-Order Filter  FilterType=Lowpass  Tc=10e-3  Ts=5e-6  Initialize=off  Vac_Init=[0.8 -25 60]  Vdc_Init=0  PlotResponse=off  param1=[1 100 0.1]
      settings: SourceProductBaseCode=PS
  To Workspace1 : ToWorkspace  VariableName=Pdc  SampleTime=-1
  To Workspace2 : ToWorkspace  VariableName=Pdc1  SampleTime=-1
  tag scope: Pdc=global
  wires:
  Pdc/1 -> [Pdc], To Workspace1/1, LPF vq7/1
  LPF vq7/1 -> To Workspace2/1

== system microgrid/Subsystem/Subsystem4 ==
  Ppv : Inport
  LPF vq7 : powerlib_extras/Discrete  Control Blocks/Discrete 1st-Order Filter  FilterType=Lowpass  Tc=10e-3  Ts=5e-6  Initialize=off  Vac_Init=[0.8 -25 60]  Vdc_Init=0  PlotResponse=off  param1=[1 100 0.1]
      settings: SourceProductBaseCode=PS
  To Workspace1 : ToWorkspace  VariableName=Ppv  SampleTime=-1
  To Workspace2 : ToWorkspace  VariableName=Ppv1  SampleTime=-1
  tag scope: Ppv=global
  wires:
  Ppv/1 -> [Ppv], To Workspace1/1, LPF vq7/1
  LPF vq7/1 -> To Workspace2/1

== system microgrid/Subsystem/Subsystem5 ==
  Pbat : Inport
  LPF vq7 : powerlib_extras/Discrete  Control Blocks/Discrete 1st-Order Filter  FilterType=Lowpass  Tc=10e-3  Ts=5e-6  Initialize=off  Vac_Init=[0.8 -25 60]  Vdc_Init=0  PlotResponse=off  param1=[1 100 0.1]
      settings: SourceProductBaseCode=PS
  To Workspace1 : ToWorkspace  VariableName=Pbat  SampleTime=-1
  To Workspace2 : ToWorkspace  VariableName=Pbat1  SampleTime=-1
  tag scope: Pbat=global
  wires:
  Pbat/1 -> [Pbat], To Workspace1/1, LPF vq7/1
  LPF vq7/1 -> To Workspace2/1

== system microgrid/Subsystem/Subsystem6 ==
  Vab_rms : Inport
  To Workspace1 : ToWorkspace  VariableName=Vab_rms  SampleTime=-1
  tag scope: Vab_rms=global
  wires:
  Vab_rms/1 -> To Workspace1/1, [Vab_rms]

== system microgrid/Subsystem/Subsystem7 ==
  Va_rms : Inport
  To Workspace1 : ToWorkspace  VariableName=Va_rms  SampleTime=-1
  tag scope: Va_rms=global
  wires:
  Va_rms/1 -> [Va_rms], To Workspace1/1

== system microgrid/Subsystem/Subsystem8 ==
  Pdcinv : Inport
  LPF vq7 : powerlib_extras/Discrete  Control Blocks/Discrete 1st-Order Filter  FilterType=Lowpass  Tc=10e-3  Ts=5e-6  Initialize=off  Vac_Init=[0.8 -25 60]  Vdc_Init=0  PlotResponse=off  param1=[1 100 0.1]
      settings: SourceProductBaseCode=PS
  To Workspace1 : ToWorkspace  VariableName=Pdcinv  SampleTime=-1
  To Workspace2 : ToWorkspace  VariableName=Pdcinv1  SampleTime=-1
  tag scope: Pdcinv=global
  wires:
  Pdcinv/1 -> [Pdcinv], To Workspace1/1, LPF vq7/1
  LPF vq7/1 -> To Workspace2/1

== system microgrid/Subsystem/Subsystem9 ==
  Mux1 : Mux  Inputs=3
  Iabc : Outport
  wires:
  [Ia] -> Mux1/1
  [Ib] -> Mux1/2
  [Ic] -> Mux1/3
  Mux1/1 -> Iabc/1

== system microgrid/Bidirectional DC//DC Converter/Battery Converter Control/PI 2 ==
  e : Inport
  Gain1 : Gain  Gain=mg.Kp_i_bat
  Gain2 : Gain  Gain=mg.Ki_i_bat
  Integrator : Integrator  LimitOutput=on  UpperSaturationLimit=mg.Dbat_trim  LowerSaturationLimit=-mg.Dbat_trim
  Saturation : Saturate  UpperLimit=mg.Dbat_trim  LowerLimit=-mg.Dbat_trim
  Sum1 : Sum  Inputs=|++
  " " : Outport
  wires:
  Sum1/1 -> Saturation/1
  Integrator/1 -> Sum1/2
  Gain1/1 -> Sum1/1
  e/1 -> Gain2/1, Gain1/1
  Gain2/1 -> Integrator/1
  Saturation/1 -> " "/1

== system microgrid/Bidirectional DC//DC Converter/Battery Converter Control/Subsystem2 ==
  Ibat_ref : Inport
  LPF vq6 : powerlib_extras/Discrete  Control Blocks/Discrete 1st-Order Filter  FilterType=Lowpass  Tc=10e-3  Ts=5e-6  Initialize=off  Vac_Init=[0.8 -25 60]  Vdc_Init=0  PlotResponse=off  param1=[1 100 0.1]
      settings: SourceProductBaseCode=PS
  To Workspace1 : ToWorkspace  VariableName=Ibat_ref  SampleTime=-1
  tag scope: Ibat_ref=global
  wires:
  LPF vq6/1 -> To Workspace1/1, [Ibat_ref]
  Ibat_ref/1 -> LPF vq6/1

== system microgrid/Bidirectional DC//DC Converter/Battery Converter Control/Subsystem3 ==
  ILbat : Inport
  LPF vq6 : powerlib_extras/Discrete  Control Blocks/Discrete 1st-Order Filter  FilterType=Lowpass  Tc=10e-3  Ts=5e-6  Initialize=off  Vac_Init=[0.8 -25 60]  Vdc_Init=0  PlotResponse=off  param1=[1 100 0.1]
      settings: SourceProductBaseCode=PS
  To Workspace1 : ToWorkspace  VariableName=ILbat  SampleTime=-1
  wires:
  ILbat/1 -> LPF vq6/1
  LPF vq6/1 -> To Workspace1/1

== system microgrid/Bidirectional DC//DC Converter/Battery Converter Control/Subsystem4 ==
  S1 : Inport
  To Workspace1 : ToWorkspace  VariableName=S1  SampleTime=-1
  Zero-Order Hold : ZeroOrderHold  SampleTime=5e-6
  wires:
  S1/1 -> Zero-Order Hold/1
  Zero-Order Hold/1 -> To Workspace1/1

== system microgrid/Bidirectional DC//DC Converter/Battery Converter Control/Subsystem5 ==
  S2 : Inport
  To Workspace1 : ToWorkspace  VariableName=S2  SampleTime=-1
  Zero-Order Hold : ZeroOrderHold  SampleTime=5e-6
  wires:
  S2/1 -> Zero-Order Hold/1
  Zero-Order Hold/1 -> To Workspace1/1

== system microgrid/PV + Boost/Boost Converter/AC Current Sensor1 ==
  Current Sensor : fl_lib/Electrical/Electrical Sensors/Current Sensor
  PS-Simulink Converter : nesl_utility/PS-Simulink Converter  PhysicalDomain=network_engine_domain  SubClassName=ps_output  LeftPortType=input  RightPortType=output  PseudoPeriodic=off  Frequencies=[]  Unit=1  AffineConversion=off
      settings: SourceProductBaseCode=PW,SS
  Sensor dynamics : TransferFcn  Numerator=1  Denominator=[1/sensor.samplingFreq 1]
  - : PMIOPort  Side=Left
  + : PMIOPort  Port=2  Side=Right
  tag scope: IL=global
  wires:
  PS-Simulink Converter/1 -> Sensor dynamics/1
  Sensor dynamics/1 -> [IL]
  connections:
  Current Sensor/RConn1 -- PS-Simulink Converter/LConn1
  +/RConn1 -- Current Sensor/LConn1
  Current Sensor/RConn2 -- -/RConn1

== system microgrid/PV + Boost/PV Control/Constant Voltage ==
  note: Current controller
  note: Voltage Control
  Vconst : Inport
  Vpv : Inport  Port=2
  "Vo " : Inport  Port=3
  IL : Inport  Port=4
  Enable : EnablePort  StatesWhenEnabling=reset
  Constant : Constant  Value=mg.Vpv_ctrl_ref
  Current control : Subsystem
  Divide : Product  Inputs=*/
  PWM Generator : eePwmGenerator/PWM Generator  CarrCount=Up  Tper=1/solarPlant.converterSwitchingFrequency  Tdelay=0  Ts=1/(10*solarPlant.converterSwitchingFrequency)
  Rate Transition1 : RateTransition  OutPortSampleTime=1/(10*solarPlant.converterSwitchingFrequency)
  Saturation : Saturate  UpperLimit=1  LowerLimit=0
  Subtract : Sum  Inputs=+-
  Sum : Sum  Inputs=|+-
  Sum2 : Sum  Inputs=|+-
  Sum3 : Sum  Inputs=|+-
  Switch : Switch  Criteria=u2 > Threshold  Threshold=mg.Vpv_ctrl_ref*0.7
  Voltage control : Subsystem
  G : Outport
  wires:
  Switch/1 -> Divide/2, Subtract/2
  Constant/1 -> Switch/3
  "Vo "/1 -> Sum/2
  Vconst/1 -> Switch/2, Switch/1, Sum/1
  Divide/1 -> Sum3/2
  PWM Generator/1 -> G/1
  Rate Transition1/1 -> PWM Generator/1
  Sum3/1 -> Saturation/1
  Vpv/1 -> Subtract/1
  Sum/1 -> Voltage control/1(e)
  Voltage control/1(u) -> Sum2/1
  Current control/1(u) -> Sum3/1
  Sum2/1 -> Current control/1(e)
  Subtract/1 -> Divide/1
  Saturation/1 -> Rate Transition1/1  "set"
  IL/1 -> Sum2/2

== system microgrid/PV + Boost/PV Control/Maximum Power Point ==
  "IL " : Inport
  "Vo " : Inport  Port=2
  Vpv : Inport  Port=3
  Ipv : Inport  Port=4
  Enable : EnablePort  StatesWhenEnabling=reset
  MPPT : Subsystem
  MPPT Subsystem : Subsystem  TreatAsAtomicUnit=on
  Rate Transition : RateTransition  OutPortSampleTime=solarPlant.timeMPPT
  ZOH/4 : ZeroOrderHold  SampleTime=solarPlant.timeMPPT
  Gmpp : Outport
  Vmpp : Outport  Port=2
  wires:
  ZOH/4/1 -> MPPT/2(Vpv)
  Rate Transition/1 -> MPPT/1(Ipv)
  MPPT/1(Vmpp) -> Vmpp/1, MPPT Subsystem/1(VpvRef)
  "Vo "/1 -> MPPT Subsystem/4("Vo ")
  Ipv/1 -> Rate Transition/1
  Vpv/1 -> MPPT Subsystem/2(Vpv), ZOH/4/1
  MPPT Subsystem/1(G) -> Gmpp/1
  "IL "/1 -> MPPT Subsystem/3(IL)

== system microgrid/PV + Boost/PV Control/PV Mode ==
  PV Mode1 : Constant
  PV Mode2 : Constant  Value=0
  PV Mode3 : Constant
  Switch : Switch  Criteria=u2 > Threshold  Threshold=0.5
  Switch1 : Switch  Criteria=u2 > Threshold  Threshold=0.5
  log pvEnMPPT : ToWorkspace  VariableName=pvEnMPPT  SaveFormat=Structure With Time  SampleTime=-1
      settings: Decimation=20
  log pvEnVctrl : ToWorkspace  VariableName=pvEnVctrl  SaveFormat=Structure With Time  SampleTime=-1
      settings: Decimation=20
  MPPT : Outport
  VoltCtrl : Outport  Port=2
  wires:
  PV Mode1/1 -> Switch/1
  PV Mode2/1 -> Switch1/1, Switch/3
  Switch/1 -> MPPT/1, log pvEnMPPT/1
  PV Mode3/1 -> Switch1/3
  Switch1/1 -> VoltCtrl/1, log pvEnVctrl/1
  [pvMode] -> Switch/2, Switch1/2

== system microgrid/PV + Boost/Solar Plant/Solar Panel ==
  Current-Controlled Current Source : fl_lib/Electrical/Electrical Sources/Current-Controlled Current Source  K=-1*(solarPanel.numParallelCell-1)  i1_specify=off  i1_priority=None  i1=0 A  i1_nominal_specify=off  i1_nominal_unit=A  i1_nominal_value=1  i2_specify=off  i2_priority=None  i2=0 A  i2_nominal_specify=off  i2_nominal_unit=A  i2_nominal_value=1
      settings: SourceProductBaseCode=SS  InternalSimscapePortConfiguration="{\"Bottom\":[],\"Left\":[{\"id\":\"p1\",\"label\":\"+\",\"type\":\"foundation.electrical.electrical\"},{\"id\":\"head\",\"label\":\"\",\"type\":\"foundation.electrical.electrical\"}],\"Right\":[{\"id\":\"n1\",\"label\":\"-\",\"type\":\"foundation.electrical.electrical\"},{\"id\":\"tail\",\"label\":\"\",\"type\":\"foundation.electrical.electrical\"}],\"Top\":[]}"
  Solar Cell : ee_lib/Sources/Solar Cell  prm=1  Isc=solarPanel.shortCircuitCurrentPV/solarPanel.numParallelCell A  Voc=solarPanel.openCircuitVoltagePV/solarPanel.numSeriesCell V  Is=1e-6 A  Is2=0 A  Iph=7.34 A  Ir0=solarPanel.irradianceMeasurement W/m^2  ec=solarPanel.qualityFactor  N2=2  Rs=solarPanel.seriesResistance Ohm  Rp=inf Ohm  N_series=solarPanel.numSeriesCell-1  N_parallel=1  TIPH1=solarPanel.currentTemperatureCoeff 1/K  EG=1.11 eV  TXIS1=solarPanel.temperatureExponent  TXIS2=3  TRS1=0  TRP1=0  Tmeas=solarPanel.temperatureMeasurement degC  TFIXED=environment.temperature degC  thermal_mass=100 J/K  initial_temperature=25 degC
      settings: SourceProductBaseCode=PS
  Ir : PMIOPort  Side=Left
  + : PMIOPort  Port=2  Side=Right
  - : PMIOPort  Port=3  Side=Right
  connections:
  Current-Controlled Current Source/LConn2 -- -/RConn1 -- Solar Cell/RConn1
  Ir/RConn1 -- Solar Cell/LConn1
  Current-Controlled Current Source/LConn1 -- Solar Cell/LConn2
  Current-Controlled Current Source/RConn1 -- Current-Controlled Current Source/RConn2 -- +/RConn1

== system microgrid/Subsystem/Inverter Control Measurements/Subsystem1 ==
  vd_ref : Inport
  To Workspace1 : ToWorkspace  VariableName=vd_ref  SampleTime=-1
  Zero-Order Hold1 : ZeroOrderHold  SampleTime=5e-6
  wires:
  vd_ref/1 -> Zero-Order Hold1/1
  Zero-Order Hold1/1 -> To Workspace1/1

== system microgrid/Subsystem/Inverter Control Measurements/Subsystem10 ==
  f_ref : Inport
  To Workspace1 : ToWorkspace  VariableName=f_ref  SampleTime=-1
  Zero-Order Hold1 : ZeroOrderHold  SampleTime=5e-6
  wires:
  f_ref/1 -> Zero-Order Hold1/1
  Zero-Order Hold1/1 -> To Workspace1/1

== system microgrid/Subsystem/Inverter Control Measurements/Subsystem11 ==
  theta : Inport
  To Workspace1 : ToWorkspace  VariableName=theta  SampleTime=-1
  Zero-Order Hold1 : ZeroOrderHold  SampleTime=5e-6
  wires:
  theta/1 -> Zero-Order Hold1/1
  Zero-Order Hold1/1 -> To Workspace1/1

== system microgrid/Subsystem/Inverter Control Measurements/Subsystem12 ==
  m_index : Inport
  To Workspace1 : ToWorkspace  VariableName=m_index  SampleTime=-1
  Zero-Order Hold1 : ZeroOrderHold  SampleTime=5e-6
  wires:
  m_index/1 -> Zero-Order Hold1/1
  Zero-Order Hold1/1 -> To Workspace1/1

== system microgrid/Subsystem/Inverter Control Measurements/Subsystem13 ==
  pulses : Inport
  To Workspace1 : ToWorkspace  VariableName=pulses  SampleTime=-1
  Zero-Order Hold1 : ZeroOrderHold  SampleTime=5e-6
  wires:
  pulses/1 -> Zero-Order Hold1/1
  Zero-Order Hold1/1 -> To Workspace1/1

== system microgrid/Subsystem/Inverter Control Measurements/Subsystem2 ==
  vq_ref : Inport
  To Workspace1 : ToWorkspace  VariableName=vq_ref  SampleTime=-1
  Zero-Order Hold1 : ZeroOrderHold  SampleTime=5e-6
  wires:
  vq_ref/1 -> Zero-Order Hold1/1
  Zero-Order Hold1/1 -> To Workspace1/1

== system microgrid/Subsystem/Inverter Control Measurements/Subsystem3 ==
  vd : Inport
  To Workspace1 : ToWorkspace  VariableName=vd  SampleTime=-1
  Zero-Order Hold1 : ZeroOrderHold  SampleTime=5e-6
  wires:
  vd/1 -> Zero-Order Hold1/1
  Zero-Order Hold1/1 -> To Workspace1/1

== system microgrid/Subsystem/Inverter Control Measurements/Subsystem4 ==
  vq : Inport
  To Workspace1 : ToWorkspace  VariableName=vq  SampleTime=-1
  Zero-Order Hold1 : ZeroOrderHold  SampleTime=5e-6
  wires:
  vq/1 -> Zero-Order Hold1/1
  Zero-Order Hold1/1 -> To Workspace1/1

== system microgrid/Subsystem/Inverter Control Measurements/Subsystem5 ==
  id_ref : Inport
  To Workspace1 : ToWorkspace  VariableName=id_ref  SampleTime=-1
  Zero-Order Hold1 : ZeroOrderHold  SampleTime=5e-6
  wires:
  id_ref/1 -> Zero-Order Hold1/1
  Zero-Order Hold1/1 -> To Workspace1/1

== system microgrid/Subsystem/Inverter Control Measurements/Subsystem6 ==
  id : Inport
  To Workspace1 : ToWorkspace  VariableName=id  SampleTime=-1
  Zero-Order Hold1 : ZeroOrderHold  SampleTime=5e-6
  wires:
  id/1 -> Zero-Order Hold1/1
  Zero-Order Hold1/1 -> To Workspace1/1

== system microgrid/Subsystem/Inverter Control Measurements/Subsystem7 ==
  iq_ref : Inport
  To Workspace1 : ToWorkspace  VariableName=iq_ref  SampleTime=-1
  Zero-Order Hold1 : ZeroOrderHold  SampleTime=5e-6
  wires:
  iq_ref/1 -> Zero-Order Hold1/1
  Zero-Order Hold1/1 -> To Workspace1/1

== system microgrid/Subsystem/Inverter Control Measurements/Subsystem8 ==
  iq : Inport
  To Workspace1 : ToWorkspace  VariableName=iq  SampleTime=-1
  Zero-Order Hold1 : ZeroOrderHold  SampleTime=5e-6
  wires:
  iq/1 -> Zero-Order Hold1/1
  Zero-Order Hold1/1 -> To Workspace1/1

== system microgrid/Subsystem/Inverter Control Measurements/Subsystem9 ==
  Vabc_ref : Inport
  To Workspace1 : ToWorkspace  VariableName=Vabc_ref  SampleTime=-1
  Zero-Order Hold1 : ZeroOrderHold  SampleTime=5e-6
  wires:
  Vabc_ref/1 -> Zero-Order Hold1/1
  Zero-Order Hold1/1 -> To Workspace1/1

== system microgrid/Subsystem/Inverter Control Measurements3/PLL ==
  Vabc : Inport
  Demux : Demux  Outputs=2
  Integrator : Integrator
  PI : Subsystem
  Subsystem3 : Subsystem
  Terminator : Terminator
  abc  - d/q : Subsystem
  wires:
  Vabc/1 -> abc  - d/q/1(abc)
  Integrator/1 -> abc  - d/q/2(tita)
  PI/1(w) -> Integrator/1, Subsystem3/1(wabc)
  Demux/2 -> PI/1(e)
  abc  - d/q/1(d/q) -> Demux/1
  Demux/1 -> Terminator/1

== system microgrid/Subsystem/Inverter Control Measurements3/Subsystem ==
  LPF vq2 : powerlib_extras/Discrete  Control Blocks/Discrete 1st-Order Filter  FilterType=Lowpass  Tc=10e-3  Ts=5e-6  Initialize=off  Vac_Init=[0.8 -25 60]  Vdc_Init=0  PlotResponse=off  param1=[1 100 0.1]
      settings: SourceProductBaseCode=PS
  LPF vq3 : powerlib_extras/Discrete  Control Blocks/Discrete 1st-Order Filter  FilterType=Lowpass  Tc=10e-3  Ts=5e-6  Initialize=off  Vac_Init=[0.8 -25 60]  Vdc_Init=0  PlotResponse=off  param1=[1 100 0.1]
      settings: SourceProductBaseCode=PS
  LPF vq4 : powerlib_extras/Discrete  Control Blocks/Discrete 1st-Order Filter  FilterType=Lowpass  Tc=10e-3  Ts=5e-6  Initialize=off  Vac_Init=[0.8 -25 60]  Vdc_Init=0  PlotResponse=off  param1=[1 100 0.1]
      settings: SourceProductBaseCode=PS
  Mux : Mux  Inputs=3
  Vabc : Outport
  wires:
  [Vab] -> LPF vq2/1
  [Vbc] -> LPF vq3/1
  [Vca] -> LPF vq4/1
  LPF vq2/1 -> Mux/1
  LPF vq3/1 -> Mux/2
  LPF vq4/1 -> Mux/3
  Mux/1 -> Vabc/1

== system microgrid/Subsystem/Load Power Calculation/Subsystem1 ==
  Qacload : Inport
  LPF vq7 : powerlib_extras/Discrete  Control Blocks/Discrete 1st-Order Filter  FilterType=Lowpass  Tc=10e-3  Ts=5e-6  Initialize=off  Vac_Init=[0.8 -25 60]  Vdc_Init=0  PlotResponse=off  param1=[1 100 0.1]
      settings: SourceProductBaseCode=PS
  To Workspace1 : ToWorkspace  VariableName=Qacload  SampleTime=-1
  To Workspace2 : ToWorkspace  VariableName=Qacload1  SampleTime=-1
  Zero-Order Hold : ZeroOrderHold  SampleTime=5e-6
  tag scope: Qacload=global
  wires:
  Qacload/1 -> Zero-Order Hold/1
  Zero-Order Hold/1 -> [Qacload], To Workspace2/1, LPF vq7/1
  LPF vq7/1 -> To Workspace1/1

== system microgrid/Subsystem/Load Power Calculation/Subsystem2 ==
  Pload : Inport
  LPF vq7 : powerlib_extras/Discrete  Control Blocks/Discrete 1st-Order Filter  FilterType=Lowpass  Tc=10e-3  Ts=5e-6  Initialize=off  Vac_Init=[0.8 -25 60]  Vdc_Init=0  PlotResponse=off  param1=[1 100 0.1]
      settings: SourceProductBaseCode=PS
  To Workspace1 : ToWorkspace  VariableName=Pacload  SampleTime=-1
  To Workspace2 : ToWorkspace  VariableName=Pacload1  SampleTime=-1
  Zero-Order Hold : ZeroOrderHold  SampleTime=5e-6
  tag scope: Pacload=global
  wires:
  Pload/1 -> Zero-Order Hold/1
  Zero-Order Hold/1 -> [Pacload], To Workspace2/1, LPF vq7/1
  LPF vq7/1 -> To Workspace1/1
